simulink model "wahadlosprezyna"  (R2024b)
settings: Solver=ode4  StartTime=0.0  StopTime=100  FixedStep=2^-6  RelTol=1e-3
settings Model: Creator=kg53848  LastModifiedBy=kg53848

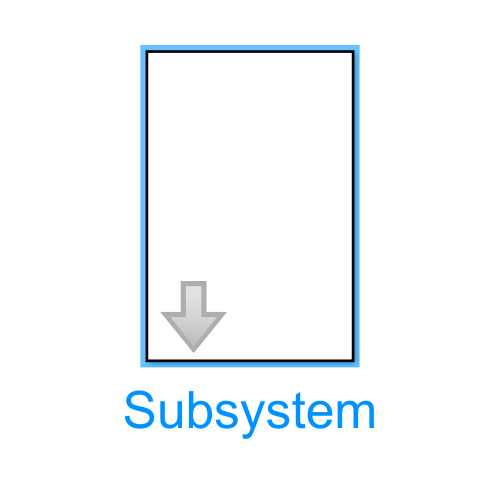
[thumbnail: Simulink's stored preview of the top-level diagram]
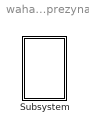
== system wahadlosprezyna ==
  Subsystem : Subsystem  mask{g=9.81, l=1.5, m=3, k=5, r0=2, r_0=1, theta0=45, theta_0=12}
      mask prompts: g "przysp"; l "dlugosc"; m "masa"; k "wspol"

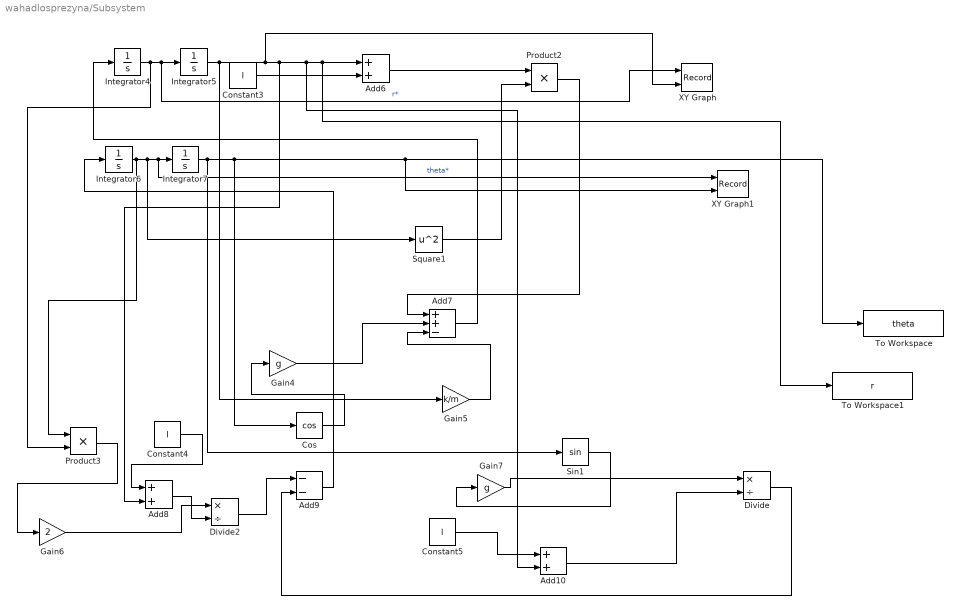
== system wahadlosprezyna/Subsystem ==
  Add10 : Sum
  Add6 : Sum
  Add7 : Sum  Inputs=++-
  Add8 : Sum
  Add9 : Sum  Inputs=--
  Constant3 : Constant  Value=l
  Constant4 : Constant  Value=l
  Constant5 : Constant  Value=l
  Cos : Trigonometry  Operator=cos
  Divide : Product  Inputs=*/
  Divide2 : Product  Inputs=*/
  Gain4 : Gain  Gain=g
  Gain5 : Gain  Gain=k/m
  Gain6 : Gain  Gain=2
  Gain7 : Gain  Gain=g
  Integrator4 : Integrator  InitialCondition=1
  Integrator5 : Integrator  InitialCondition=2
  Integrator6 : Integrator  InitialCondition=12*pi/180
  Integrator7 : Integrator  InitialCondition=45*pi/180
  Product2 : Product
  Product3 : Product
  Sin1 : Trigonometry
  Square1 : Math  Operator=square
  To Workspace : ToWorkspace  VariableName=theta  SampleTime=-1
  To Workspace1 : ToWorkspace  VariableName=r  SampleTime=-1
  XY Graph : Record  FileSettingsInternal="{\"entries\":[{\"content\":{\"excelSettings\":{\"content\":{},\"type\":\"Streamout.ExcelSettings\"}},\"type\":\"Streamout.FileSettingStorage\",\"uuid\":\"\"}],\"packageUris\":[\"http:\\/\\/schema.mathworks.com\\/mf0\\/streamout_blocks\\/R2020a\"],\"version\":\"1.0\"}"  Layout=[1 1]  SignalsInternal="{\"entries\":[{\"content\":{\"signals\":[{\"content\":{\"blockPath\":[],\"dimensions\":[1],\"domain\":\"\",\"lineColor\":\"#a2142f\",\"plots\":[ 1 ],\"port\":1,\"sid\":[\"\"],\"signalID\":1,\"signalName\":\"r*\"},\"type\":\"RecordBlkView.Signal\",\"uuid\":\"\"},{\"content\":{\"blockPath\":[],\"dimensions\":[1],\"domain\":\"\",\"lineColor\":\"#139fff\",\"plots\":[ 1 ],\"port\":2,\"sid\":[\"\"],\"signalID\":2,\"signalName\":\"Integrator5\"},\"type\":\"RecordBlkView.Signal\",\"uuid\":\"\"}]},\"type\":\"RecordBlkView.InputSignals\",\"uuid\":\"\"}],\"packageUris\":[\"http:\\/\\/schema.mathworks.com\\/mf0\\/streamout_blocks\\/R2020a\"],\"version\":\"1.0\"}"  VisualizationBindings="{\"xyplotplugin\":{\"info\":[{\"series\":[{\"bindingParametersList\":[{\"parameter\":\"X-Axis\",\"signalID\":1,\"signalName\":\"r*\"},{\"parameter\":\"Y-Axis\",\"signalID\":2,\"signalName\":\"Integrator5\"}],\"seriesID\":0}],\"subplotID\":1}]}}"  CompatibilityTag=XY
  XY Graph1 : Record  FileSettingsInternal="{\"entries\":[{\"content\":{\"excelSettings\":{\"content\":{},\"type\":\"Streamout.ExcelSettings\"}},\"type\":\"Streamout.FileSettingStorage\",\"uuid\":\"\"}],\"packageUris\":[\"http:\\/\\/schema.mathworks.com\\/mf0\\/streamout_blocks\\/R2020a\"],\"version\":\"1.0\"}"  Layout=[1 1]  SignalsInternal="{\"entries\":[{\"content\":{\"signals\":[{\"content\":{\"blockPath\":[],\"dimensions\":[1],\"domain\":\"\",\"lineColor\":\"#a2142f\",\"plots\":[ 1 ],\"port\":1,\"sid\":[\"\"],\"signalID\":1,\"signalName\":\"theta*\"},\"type\":\"RecordBlkView.Signal\",\"uuid\":\"\"},{\"content\":{\"blockPath\":[],\"dimensions\":[1],\"domain\":\"\",\"lineColor\":\"#139fff\",\"plots\":[ 1 ],\"port\":2,\"sid\":[\"\"],\"signalID\":2,\"signalName\":\"Integrator7\"},\"type\":\"RecordBlkView.Signal\",\"uuid\":\"\"}]},\"type\":\"RecordBlkView.InputSignals\",\"uuid\":\"\"}],\"packageUris\":[\"http:\\/\\/schema.mathworks.com\\/mf0\\/streamout_blocks\\/R2020a\"],\"version\":\"1.0\"}"  VisualizationBindings="{\"xyplotplugin\":{\"info\":[{\"series\":[{\"bindingParametersList\":[{\"parameter\":\"X-Axis\",\"signalID\":1,\"signalName\":\"theta*\"},{\"parameter\":\"Y-Axis\",\"signalID\":2,\"signalName\":\"Integrator7\"}],\"seriesID\":0}],\"subplotID\":1}]}}"  CompatibilityTag=XY
  wires:
  Integrator4/1 -> Product3/2, XY Graph/1, Integrator5/1  "r*"
  Integrator6/1 -> Product3/1, Square1/1, XY Graph1/1, Integrator7/1  "theta*"
  Constant3/1 -> Add6/2
  Integrator5/1 -> Gain5/1, XY Graph/2, Add8/2, Add10/2, To Workspace1/1, Add6/1
  Square1/1 -> Product2/2
  Add6/1 -> Product2/1
  Integrator7/1 -> Sin1/1, To Workspace/1, XY Graph1/2, Cos/1
  Cos/1 -> Gain4/1
  Product2/1 -> Add7/1
  Gain4/1 -> Add7/2
  Gain5/1 -> Add7/3
  Add7/1 -> Integrator4/1
  Product3/1 -> Gain6/1
  Constant4/1 -> Add8/1
  Add8/1 -> Divide2/2
  Gain6/1 -> Divide2/1
  Divide2/1 -> Add9/1
  Sin1/1 -> Gain7/1
  Constant5/1 -> Add10/1
  Add9/1 -> Integrator6/1
  Gain7/1 -> Divide/1
  Add10/1 -> Divide/2
  Divide/1 -> Add9/2
